simulink model "SImple_Missile_Simulation"  (R2024b)
settings: Solver=FixedStepAuto  StartTime=0.0  StopTime=25  FixedStep=1/100  RelTol=1e-3
libraries: simulink_extras x2, MISSILE_GUIDANCE_LIB2 x1
settings Model: Creator=leoni  LastModifiedBy=leoni
settings RTWCC: GPUComputeCapability=3.5

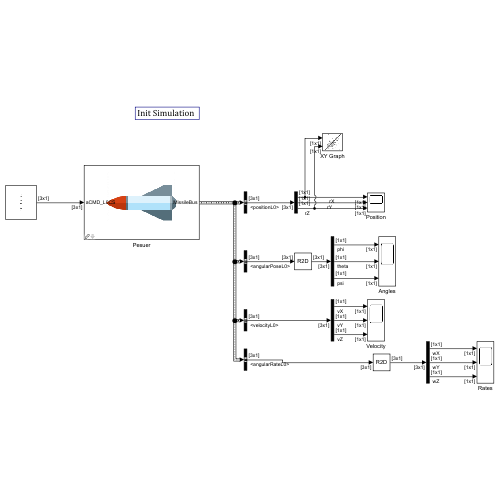
[thumbnail: Simulink's stored preview of the top-level diagram]
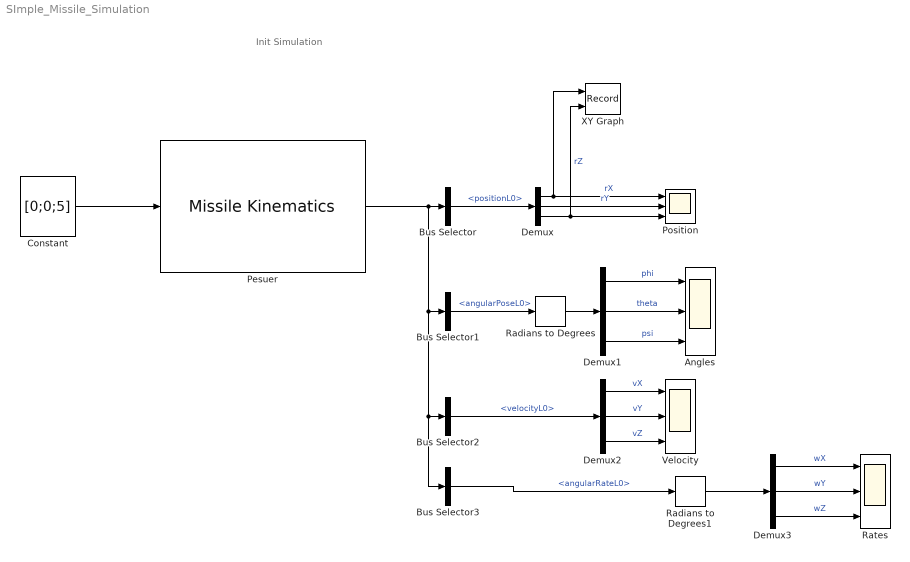
== system SImple_Missile_Simulation ==
  note: Init Simulation
  Angles : Scope  NumInputPorts=3
  Bus Selector : BusSelector  OutputSignals=positionL0
  Bus Selector1 : BusSelector  OutputSignals=angularPoseL0
  Bus Selector2 : BusSelector  OutputSignals=velocityL0
  Bus Selector3 : BusSelector  OutputSignals=angularRateL0
  Constant : Constant  Value=[0;0;5]  VectorParams1D=off
  Demux{,1..3} (4 alike) : Demux  Outputs=3
  Pesuer : MISSILE_GUIDANCE_LIB2/Missile Kinematics  psi0_theta0_phi0=[0;15;0]  vX0=100  r0=[0;0;0]  tau_X=0  tau_YZ=0
  Position : Scope  NumInputPorts=3
  Radians to Degrees : simulink_extras/Transformations/Radians to Degrees
  Radians to Degrees1 : simulink_extras/Transformations/Radians to Degrees
  Rates : Scope  NumInputPorts=3
  Velocity : Scope  NumInputPorts=3
  XY Graph : Record  FileSettingsInternal="{\"entries\":[{\"content\":{\"excelSettings\":{\"content\":{},\"type\":\"Streamout.ExcelSettings\"}},\"type\":\"Streamout.FileSettingStorage\",\"uuid\":\"\"}],\"packageUris\":[\"http:\\/\\/schema.mathworks.com\\/mf0\\/streamout_blocks\\/R2020a\"],\"version\":\"1.0\"}"  Layout=[1 1]  SignalsInternal="{\"entries\":[{\"content\":{\"signals\":[{\"content\":{\"blockPath\":[],\"dimensions\":[1,1],\"domain\":\"\",\"lineColor\":\"#a2142f\",\"plots\":[ 1 ],\"port\":1,\"sid\":[\"\"],\"signalID\":1,\"signalName\":\"rX\"},\"type\":\"RecordBlkView.Signal\",\"uuid\":\"\"},{\"content\":{\"blockPath\":[],\"dimensions\":[1,1],\"domain\":\"\",\"lineColor\":\"#139fff\",\"plots\":[ 1 ],\"port\":2,\"sid\":[\"\"],\"signalID\":2,\"signalName\":\"rZ\"},\"type\":\"RecordBlkView.Signal\",\"uuid\":\"\"}]},\"type\":\"RecordBlkView.InputSignals\",\"uuid\":\"\"}],\"packageUris\":[\"http:\\/\\/schema.mathworks.com\\/mf0\\/streamout_blocks\\/R2020a\"],\"version\":\"1.0\"}"  VisualizationBindings="{\"xyplotplugin\":{\"info\":[{\"series\":[{\"bindingParametersList\":[{\"parameter\":\"X-Axis\",\"signalID\":1,\"signalName\":\"rX\"},{\"parameter\":\"Y-Axis\",\"signalID\":2,\"signalName\":\"rZ\"}],\"seriesID\":0}],\"subplotID\":1}]}}"  CompatibilityTag=XY
  wires:
  Constant/1 -> Pesuer/1
  Pesuer/1 -> Bus Selector3/1, Bus Selector2/1, Bus Selector1/1, Bus Selector/1
  Bus Selector/1 -> Demux/1  "<positionL0>"
  Demux/1 -> XY Graph/1, Position/1  "rX"
  Demux/2 -> Position/2  "rY"
  Demux/3 -> XY Graph/2, Position/3  "rZ"
  Bus Selector1/1 -> Radians to Degrees/1  "<angularPoseL0>"
  Demux1/2 -> Angles/2  "theta"
  Radians to Degrees/1 -> Demux1/1
  Bus Selector2/1 -> Demux2/1  "<velocityL0>"
  Demux2/1 -> Velocity/1  "vX"
  Demux2/2 -> Velocity/2  "vY"
  Demux2/3 -> Velocity/3  "vZ"
  Bus Selector3/1 -> Radians to Degrees1/1  "<angularRateL0>"
  Radians to Degrees1/1 -> Demux3/1
  Demux3/1 -> Rates/1  "wX"
  Demux3/2 -> Rates/2  "wY"
  Demux3/3 -> Rates/3  "wZ"
  Demux1/1 -> Angles/1  "phi"
  Demux1/3 -> Angles/3  "psi"
